simulink model "realim_estados_pd"  (R2015a)
settings: Solver=ode45  StartTime=0.0  StopTime=10  RelTol=1e-3
values from neighbouring files (symbols this model uses):
  a = [0 1;0 0]    [ejemplo_jury.m]    (also in observer_minimum.m = [0 1;0 -1]; realim_state_pd.m = [0 1;0 -1])
  b = [0;1]    [ejemplo_jury.m]    (also in observer_minimum.m = [0; 10]; realim_state_pd.m = [0; 10])
  c = [1 0]    [ejemplo_jury.m]    (also in observer_minimum.m; realim_state_pd.m)
  d = 0    [ejemplo_jury.m]    (also in observer_minimum.m; realim_state_pd.m)
  k = 1    [ejemplo_jury.m]    (also in observer_minimum.m = [0.8 0.3]; realim_state_pd.m = [0.8 0.3])
  k1 = 2.39    [ejemplo_jury.m]    (also in observer_minimum.m = [8.8 2.3]; realim_state_pd.m = [8.8 2.3])
  k2 = 16    [observer_minimum.m]    (also in realim_state_pd.m)
  kder = 0.3    [observer_minimum.m]    (also in realim_state_pd.m)
  kp = 0.625    [controlador_digital.m]    (also in observer_minimum.m = 0.8; realim_state_pd.m = 0.8)
libraries: cstblocks x1
settings Model: Creator=Jose Roldan  LastModifiedBy=Jose Roldan

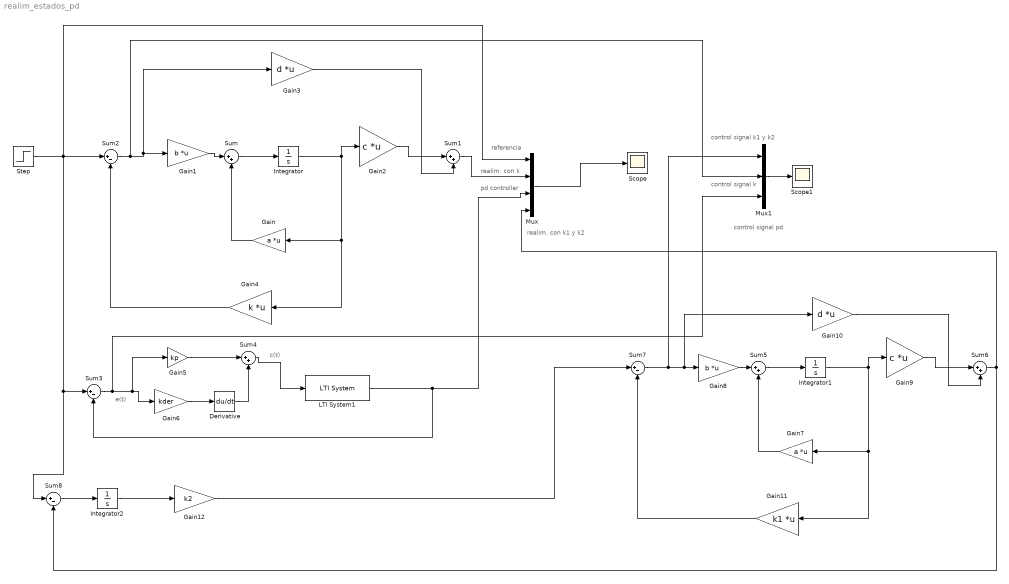
== system realim_estados_pd ==
  note: control signal pd
  note: control signal k1 y k2
  note: control signal k
  note: realim. con k1 y k2
  note: pd controller
  note: realim. con k
  note: referencia
  note: c(t)
  note: e(t)
  Derivative : Derivative
  Gain : Gain  Gain=a  Multiplication=Matrix(K*u)
  Gain1 : Gain  Gain=b  Multiplication=Matrix(K*u)
  Gain10 : Gain  Gain=d  Multiplication=Matrix(K*u)
  Gain11 : Gain  Gain=k1  Multiplication=Matrix(K*u)
  Gain12 : Gain  Gain=k2
  Gain2 : Gain  Gain=c  Multiplication=Matrix(K*u)
  Gain3 : Gain  Gain=d  Multiplication=Matrix(K*u)
  Gain4 : Gain  Gain=k  Multiplication=Matrix(K*u)
  Gain5 : Gain  Gain=kp
  Gain6 : Gain  Gain=kder
  Gain7 : Gain  Gain=a  Multiplication=Matrix(K*u)
  Gain8 : Gain  Gain=b  Multiplication=Matrix(K*u)
  Gain9 : Gain  Gain=c  Multiplication=Matrix(K*u)
  Integrator : Integrator
  Integrator1 : Integrator
  Integrator2 : Integrator
  LTI System1 : cstblocks/LTI System  sys=G  IC=[]
  Mux : Mux
  Mux1 : Mux  Inputs=3
  Scope : Scope
  Scope1 : Scope
  Step : Step  SampleTime=0
  Sum{,1,4..6} (5 alike) : Sum  Inputs=|++
  Sum{2..3,7..8} (4 alike) : Sum  Inputs=|+-
  wires:
  Step/1 -> Sum8/1, Sum3/1, Mux/1, Sum2/1
  Sum2/1 -> Mux1/2, Gain3/1, Gain1/1
  Gain1/1 -> Sum/1
  Sum/1 -> Integrator/1
  Integrator/1 -> Gain4/1, Gain/1, Gain2/1
  Gain2/1 -> Sum1/1
  Gain3/1 -> Sum1/2
  Gain/1 -> Sum/2
  Gain4/1 -> Sum2/2
  Sum1/1 -> Mux/2
  LTI System1/1 -> Sum3/2, Mux/3
  Sum4/1 -> LTI System1/1
  Sum3/1 -> Mux1/3, Gain5/1, Gain6/1
  Gain6/1 -> Derivative/1
  Derivative/1 -> Sum4/2
  Gain5/1 -> Sum4/1
  Sum7/1 -> Mux1/1, Gain10/1, Gain8/1
  Gain8/1 -> Sum5/1
  Sum5/1 -> Integrator1/1
  Integrator1/1 -> Gain11/1, Gain7/1, Gain9/1
  Gain9/1 -> Sum6/1
  Gain10/1 -> Sum6/2
  Gain7/1 -> Sum5/2
  Gain11/1 -> Sum7/2
  Sum6/1 -> Sum8/2, Mux/4
  Mux/1 -> Scope/1
  Sum8/1 -> Integrator2/1
  Integrator2/1 -> Gain12/1
  Gain12/1 -> Sum7/1
  Mux1/1 -> Scope1/1
